simulink model "platoon_test"  (R2020b)
settings: Solver=VariableStepAuto  StartTime=0.0  StopTime=70.0  RelTol=1e-3
libraries: simulink x2
settings Model: Creator=Roozbeh  LastModifiedBy=Roozbeh

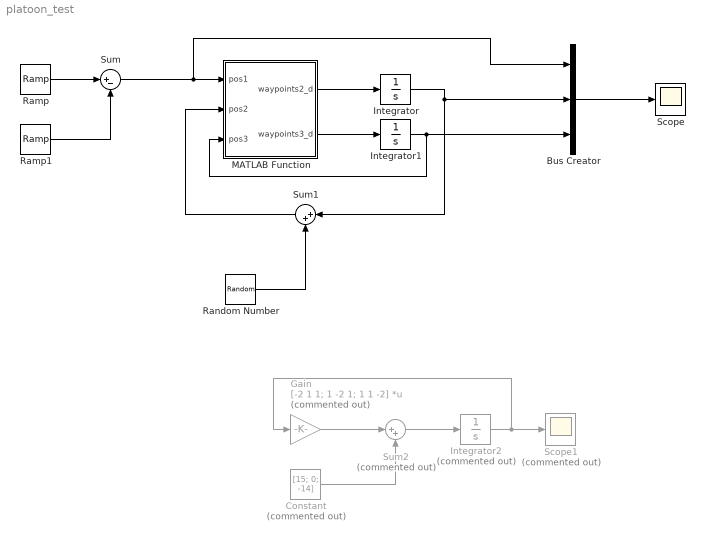
== system platoon_test ==
  Bus Creator : BusCreator  Inputs=3
  Constant : Constant  Commented=on  Value=[15; 0; -14]
  Gain : Gain  Commented=on  Gain=[-2 1 1; 1 -2 1; 1 1 -2]  Multiplication=Matrix(K*u)
  Integrator : Integrator  InitialCondition=[5 5]*0.5
  Integrator1 : Integrator  InitialCondition=[0 10]*0.95
  Integrator2 : Integrator  Commented=on  InitialCondition=[2; 5; -3]
  MATLAB Function : MATLAB Function  TreatAsAtomicUnit=on
  Ramp : simulink/Sources/Ramp  slope=[1 1]  start=15  InitialOutput=[0 0]
  Ramp1 : simulink/Sources/Ramp  slope=[1 1]  start=30  InitialOutput=[0 0]
  Random Number : RandomNumber  Variance=0  SampleTime=0.1
  Scope : Scope
  Scope1 : Scope  Commented=on
  Sum : Sum  Inputs=|+-
  Sum1 : Sum  Inputs=|++
  Sum2 : Sum  Commented=on  Inputs=|++
  wires:
  MATLAB Function/1(waypoints2_d) -> Integrator/1
  Integrator/1 -> Sum1/1, Bus Creator/2
  Bus Creator/1 -> Scope/1
  Ramp/1 -> Sum/1
  Sum/1 -> Bus Creator/1, MATLAB Function/1(pos1)
  Ramp1/1 -> Sum/2
  Integrator1/1 -> MATLAB Function/3(pos3), Bus Creator/3
  MATLAB Function/2(waypoints3_d) -> Integrator1/1
  Sum1/1 -> MATLAB Function/2(pos2)
  Random Number/1 -> Sum1/2
  Sum2/1 -> Integrator2/1
  Integrator2/1 -> Gain/1, Scope1/1
  Gain/1 -> Sum2/1
  Constant/1 -> Sum2/2

== matlab function platoon_test/MATLAB Function ==
  data: pos1 input; waypoints2_d output; pos2 input; pos3 input; waypoints3_d output
function [waypoints2_d, waypoints3_d] = fcn(pos1, pos2, pos3)

L = [-2 1 1; 1 -2 1; 1 1 -2];
F = [2 2; 0 4; 0 0];
x = [pos1(1:2)'; pos2(1:2)'; pos3(1:2)'];
xd = L*(x - F);

waypoints2_d = xd(2,:);
waypoints3_d = xd(3,:);
